simulink model "RCAM_model_Lateral"  (R2022b)
settings: Solver=VariableStepAuto  StartTime=0.0  StopTime=10.0  RelTol=1e-3
libraries: cstblocks x1
settings Model: Creator=bendr  LastModifiedBy=bendr

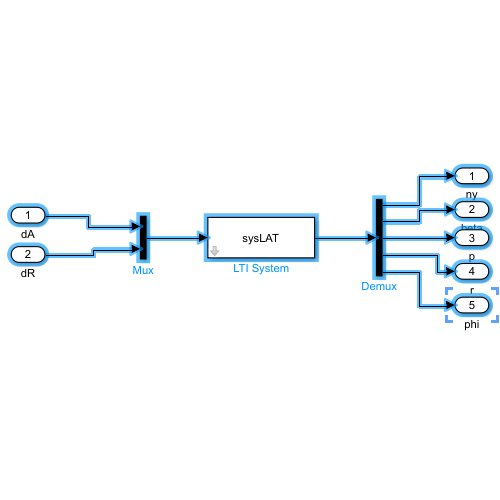
[thumbnail: Simulink's stored preview of the top-level diagram]
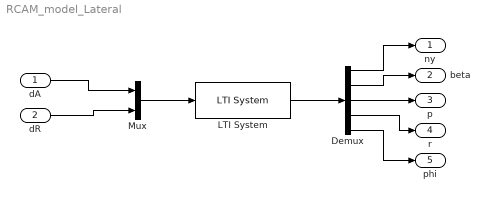
== system RCAM_model_Lateral ==
  dA : Inport
  dR : Inport  Port=2
  Demux : Demux  Outputs=5
  LTI System : cstblocks/LTI System  sys=sysLAT  IC=[]
  Mux : Mux  Inputs=2
  ny : Outport
  beta : Outport  Port=2
  p : Outport  Port=3
  r : Outport  Port=4
  phi : Outport  Port=5
  wires:
  Mux/1 -> LTI System/1
  dA/1 -> Mux/1
  dR/1 -> Mux/2
  LTI System/1 -> Demux/1
  Demux/1 -> ny/1
  Demux/2 -> beta/1
  Demux/3 -> p/1
  Demux/4 -> r/1
  Demux/5 -> phi/1
